simulink model "TVC_FSFB_model"  (R2024b)
settings: Solver=ode8  StartTime=0.0  StopTime=60  FixedStep=0.001  RelTol=1e-3
values from neighbouring files (symbols this model uses):
  A = sys_open_loop.A    [Heavy_STeVe_LQR_Testing.m]    (also in LQR_autoTuning.m)
  A_plant = [-d1  0   1 ... (first row only)    [Heavy_STeVe_LQR_Testing.m]    (also in LQR_autoTuning.m = [-d1 0 1; 0 0 1; d3 0 d4])
  B = sys_open_loop.B    [Heavy_STeVe_LQR_Testing.m]    (also in LQR_autoTuning.m)
  B_plant = [-d5 ... (first row only)    [Heavy_STeVe_LQR_Testing.m]    (also in LQR_autoTuning.m = [-d5; 0; d2])
  K_lqr = lqr(A, B, Q, R)    [Heavy_STeVe_LQR_Testing.m]    (also in LQR_autoTuning.m = K)
libraries: simulink_extras x5, aerolibactuator x2, simulink x2
settings Model: Creator=jonno  LastModifiedBy=jonno

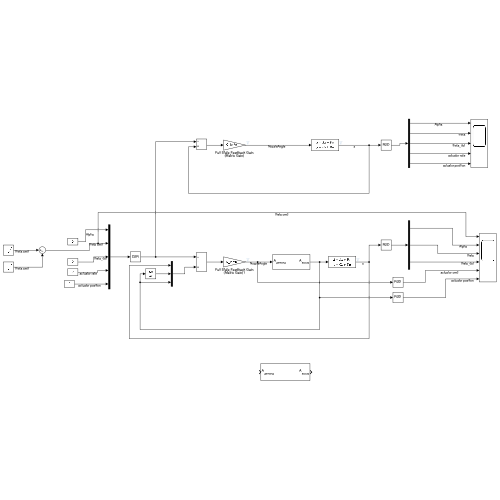
[thumbnail: Simulink's stored preview of the top-level diagram]
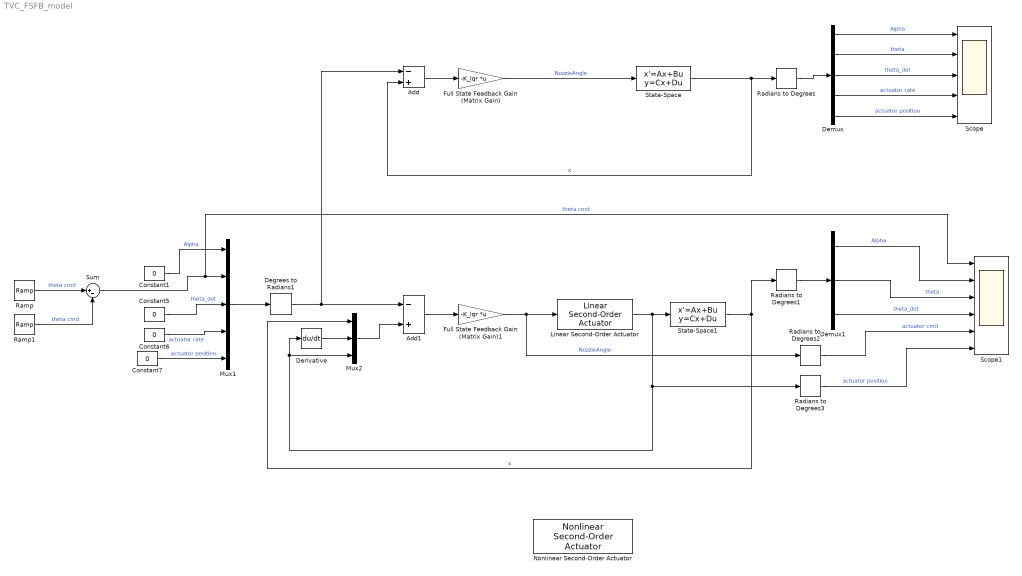
== system TVC_FSFB_model ==
  Add : Sum  Inputs=-+
  Add1 : Sum  Inputs=-+
  Constant{1,5..7} (4 alike) : Constant  Value=0
  Degrees to Radians1 : simulink_extras/Transformations/Degrees to Radians
  Demux : Demux  Outputs=5
  Demux1 : Demux  Outputs=3
  Derivative : Derivative
  Full State Feedback Gain (Matrix Gain) : Gain  Gain=-K_lqr  Multiplication=Matrix(K*u)
  Full State Feedback Gain (Matrix Gain)1 : Gain  Gain=-K_lqr  Multiplication=Matrix(K*u)
  Linear Second-Order Actuator : aerolibactuator/Linear Second-Order Actuator  wn_fin=62  z_fin=0.5858  fin_act_0=0  fin_act_vel=0
  Mux1 : Mux  Inputs=5
  Mux2 : Mux  Inputs=3
  Nonlinear Second-Order Actuator : aerolibactuator/Nonlinear Second-Order Actuator  wn_fin=62  z_fin=0.5858  fin_max=6*pi/180  fin_min=-6*pi/180  fin_maxrate=500*pi/180  fin_act_0=0  fin_act_vel=0
  Radians to Degrees{,1..3} (4 alike) : simulink_extras/Transformations/Radians to Degrees
  Ramp : simulink/Sources/Ramp  slope=0.5  start=1  InitialOutput=0
  Ramp1 : simulink/Sources/Ramp  slope=0.5  start=20  InitialOutput=0
  Scope : Scope  NumInputPorts=5
  Scope1 : Scope  NumInputPorts=6
  State-Space : StateSpace  A=A  B=B  C=eye(size(A,1))  D=zeros(size(A,1), size(B,2))  InitialCondition=[0 0 0 0 0]
  State-Space1 : StateSpace  A=A_plant  B=B_plant  C=eye(size(A_plant,1))  D=zeros(size(A_plant,1), size(B_plant,2))  InitialCondition=zeros(1, size(A_plant, 2))
  Sum : Sum  Inputs=|+-
  wires:
  Full State Feedback Gain (Matrix Gain)/1 -> State-Space/1  "NozzleAngle"
  State-Space/1 -> Radians to Degrees/1, Add/2  "x"
  Add/1 -> Full State Feedback Gain (Matrix Gain)/1
  Demux/1 -> Scope/1  "Alpha"
  Demux/3 -> Scope/3  "theta_dot"
  Demux/4 -> Scope/4  "actuator rate"
  Demux/2 -> Scope/2  "theta"
  Demux/5 -> Scope/5  "actuator position"
  Radians to Degrees/1 -> Demux/1
  Demux1/2 -> Scope1/3  "theta"
  Degrees to Radians1/1 -> Add/1, Add1/1
  Mux1/1 -> Degrees to Radians1/1
  Constant7/1 -> Mux1/5  "actuator position"
  Constant6/1 -> Mux1/4  "actuator rate"
  Sum/1 -> Scope1/1, Mux1/2  "theta cmd"
  Add1/1 -> Full State Feedback Gain (Matrix Gain)1/1
  Constant1/1 -> Mux1/1  "Alpha"
  Full State Feedback Gain (Matrix Gain)1/1 -> Linear Second-Order Actuator/1, Radians to Degrees2/1  "NozzleAngle"
  Constant5/1 -> Mux1/3  "theta_dot"
  State-Space1/1 -> Mux2/1, Radians to Degrees1/1  "x"
  Demux1/1 -> Scope1/2  "Alpha"
  Demux1/3 -> Scope1/4  "theta_dot"
  Radians to Degrees3/1 -> Scope1/6  "actuator position"
  Radians to Degrees1/1 -> Demux1/1
  Mux2/1 -> Add1/2
  Linear Second-Order Actuator/1 -> Radians to Degrees3/1, Mux2/3, Derivative/1, State-Space1/1
  Derivative/1 -> Mux2/2
  Radians to Degrees2/1 -> Scope1/5  "actuator cmd"
  Ramp/1 -> Sum/1  "theta cmd"
  Ramp1/1 -> Sum/2  "theta cmd"
